simulink model "BCM2_4"  (R2021b)
settings: Solver=FixedStepDiscrete  StartTime=0.0  StopTime=1  FixedStep=0.001  RelTol=1e-3  EnableMultiTasking=on
InitFcn:
  | mbd_mpc_consistency_checks(bdroot(gcs));
model workspace (MAT data in the model file):
  CAN_rec : Simulink.Signal (value not decoded)
  CAN_transm_stat : Simulink.Signal (value not decoded)
  CAN_trm : Simulink.Signal (value not decoded)
  DITHER_CFB0 : Simulink.Parameter (value not decoded)
  DITHER_CFB1 : Simulink.Parameter (value not decoded)
  DITHER_CFB2 : Simulink.Parameter (value not decoded)
  DITHER_EN0 : Simulink.Parameter (value not decoded)
  DITHER_EN1 : Simulink.Parameter (value not decoded)
  DITHER_EN2 : Simulink.Parameter (value not decoded)
  DITHER_SIZE0 : Simulink.Parameter (value not decoded)
  DITHER_SIZE1 : Simulink.Parameter (value not decoded)
  DITHER_SIZE2 : Simulink.Parameter (value not decoded)
  DITHER_STEP0 : Simulink.Parameter (value not decoded)
  DITHER_STEP1 : Simulink.Parameter (value not decoded)
  DITHER_STEP2 : Simulink.Parameter (value not decoded)
  DITHER_SYNC0 : Simulink.Parameter (value not decoded)
  DITHER_SYNC1 : Simulink.Parameter (value not decoded)
  DITHER_SYNC2 : Simulink.Parameter (value not decoded)
  ECUMbut : Simulink.Signal (value not decoded)
  FAULTN : Simulink.Signal (value not decoded)
  FM0 : Simulink.Parameter (value not decoded)
  FM1 : Simulink.Parameter (value not decoded)
  FM2 : Simulink.Parameter (value not decoded)
  FME : Simulink.Parameter (value not decoded)
  Fsys_M : Simulink.Parameter (value not decoded)
  Fsys_N : Simulink.Parameter (value not decoded)
  Fsys_WDEN : Simulink.Parameter (value not decoded)
  Fsys_div : Simulink.Parameter (value not decoded)
  HL0 : Simulink.Parameter (value not decoded)
  HL1 : Simulink.Parameter (value not decoded)
  HL2 : Simulink.Parameter (value not decoded)
  IDIAG0 : Simulink.Parameter (value not decoded)
  IDIAG1 : Simulink.Parameter (value not decoded)
  IDIAG2 : Simulink.Parameter (value not decoded)
  Ivalve : Simulink.Signal (value not decoded)
  KI_index0 : Simulink.Parameter (value not decoded)
  KI_index1 : Simulink.Parameter (value not decoded)
  KI_index2 : Simulink.Parameter (value not decoded)
  PWM_Period0 : Simulink.Parameter (value not decoded)
  PWM_Period1 : Simulink.Parameter (value not decoded)
  PWM_Period2 : Simulink.Parameter (value not decoded)
  RESN : Simulink.Signal (value not decoded)
  SR0 : Simulink.Parameter (value not decoded)
  SR1 : Simulink.Parameter (value not decoded)
  SR2 : Simulink.Parameter (value not decoded)
  Vparam : Simulink.Signal (value not decoded)
  block_tle : Simulink.Signal (value not decoded)
  disp : Simulink.Signal (value not decoded)
  ee_adr : Simulink.Signal (value not decoded)
  ee_en_rd : Simulink.Signal (value not decoded)
  ee_en_wr : Simulink.Signal (value not decoded)
  ee_idle : Simulink.Signal (value not decoded)
  ee_read : Simulink.Signal (value not decoded)
  ee_recv : Simulink.Signal (value not decoded)
  ee_send : Simulink.Signal (value not decoded)
  in_stats : Simulink.Signal (value not decoded)
  inputs : Simulink.Signal (value not decoded)
  light : Simulink.Signal (value not decoded)
  out_drv : Simulink.Signal (value not decoded)
  out_drv_test : Simulink.Signal (value not decoded)
  out_test_en : Simulink.Signal (value not decoded)
  recv_spi2 : Simulink.Signal (value not decoded)
  ret : Simulink.Signal (value not decoded)
  spi_rcv_tle82453 : Simulink.Signal (value not decoded)
  tle82453_Ivlv : Simulink.Signal (value not decoded)
  tle82453_err : Simulink.Signal (value not decoded)
  tle82453_reset : Simulink.Signal (value not decoded)
  wtdg_CAN : Simulink.Signal (value not decoded)
symbols that are objects in the model workspace (value not decoded): CAN_rec, CAN_transm_stat, ECUMbut, inputs, Ivalve, out_drv_test, recv_spi2, ret, SR0, tle82453_Ivlv
undefined symbols (not defined in the file or in its folder): color, LQFP
libraries: simulink x68, mbd_mpc574x_ec_toolbox x50, canmsglib x42, hdlsllib x9, commutil2 x7, etargetslib x4
(part 4 of 6)

== system BCM2_4/CAN0 Transmit buf 5-21/18FEEA2F buf = 9/18FEEA2F buf = 9 ==
  Constant4 : Constant  OutDataTypeStr=boolean
  Data Store Read : DataStoreRead  DataStoreName=CAN_rec  DataStoreElements=CAN_rec.m18FEEA2F(:)  IndexOptions=Index vector (dialog)  Indices=1  OutputSizes=1
  Data Store Write : DataStoreWrite  DataStoreName=CAN_transm_stat  DataStoreElements=CAN_transm_stat(9)  IndexOptions=Index vector (dialog)  Indices=1  OutputSizes=1
  FCAN_Send : mbd_mpc574x_ec_toolbox/Communication Blocks/CAN Blocks/FCAN_Send  Priority=2  can_instance=0  can_mode=Non-blocking  can_timeout_ms=0  can_mb_idx=9  can_extended_id=on  can_is_remote=off  can_id=18FEEA2F  show_adv_opts=on  can_fd_enable=off  can_enable_brs=off  can_fd_padding=0
      settings: SourceProductName=NXP Model-Based Design Toolbox for MPC57xx MCUs
  Width : Width  DataType=uint8
  wires:
  Data Store Read/1 -> FCAN_Send/1, Width/1
  Constant4/1 -> Data Store Write/1
  Width/1 -> FCAN_Send/2

== system BCM2_4/CAN0 Transmit buf 5-21/Tx_Complete/If Action Subsystem1 ==
  Action Port : ActionPort  ActionPortLabel=case [ 7 ]:
  Constant : Constant  Value=0  OutDataTypeStr=boolean
  Data Store Write : DataStoreWrite  DataStoreName=CAN_transm_stat  DataStoreElements=CAN_transm_stat(7)  IndexOptions=Index vector (dialog)  Indices=1  OutputSizes=1
  wires:
  Constant/1 -> Data Store Write/1

== system BCM2_4/CAN0 Transmit buf 5-21/Tx_Complete/If Action Subsystem2 ==
  Action Port : ActionPort  ActionPortLabel=default:

== system BCM2_4/CAN0 Transmit buf 5-21/Tx_Complete/If Action Subsystem3 ==
  Action Port : ActionPort  ActionPortLabel=case [ 8 ]:
  Constant : Constant  Value=0  OutDataTypeStr=boolean
  Data Store Write : DataStoreWrite  DataStoreName=CAN_transm_stat  DataStoreElements=CAN_transm_stat(8)  IndexOptions=Index vector (dialog)  Indices=1  OutputSizes=1
  wires:
  Constant/1 -> Data Store Write/1

== system BCM2_4/CAN0 Transmit buf 5-21/Tx_Complete/If Action Subsystem4 ==
  Action Port : ActionPort  ActionPortLabel=case [ 9 ]:
  Constant : Constant  Value=0  OutDataTypeStr=boolean
  Data Store Write : DataStoreWrite  DataStoreName=CAN_transm_stat  DataStoreElements=CAN_transm_stat(9)  IndexOptions=Index vector (dialog)  Indices=1  OutputSizes=1
  wires:
  Constant/1 -> Data Store Write/1

== system BCM2_4/CAN0 Transmit buf 5-21/Tx_Complete/If Action Subsystem5 ==
  Action Port : ActionPort  ActionPortLabel=case [ 10 ]:
  Constant : Constant  Value=0  OutDataTypeStr=boolean
  Data Store Write : DataStoreWrite  DataStoreName=CAN_transm_stat  DataStoreElements=CAN_transm_stat(10)  IndexOptions=Index vector (dialog)  Indices=1  OutputSizes=1
  wires:
  Constant/1 -> Data Store Write/1

== system BCM2_4/CAN0 Transmit buf 5-21/Tx_Complete/If Action Subsystem6 ==
  Action Port : ActionPort  ActionPortLabel=case [ 11 ]:
  Constant : Constant  Value=0  OutDataTypeStr=boolean
  Data Store Write : DataStoreWrite  DataStoreName=CAN_transm_stat  DataStoreElements=CAN_transm_stat(11)  IndexOptions=Index vector (dialog)  Indices=1  OutputSizes=1
  wires:
  Constant/1 -> Data Store Write/1

== system BCM2_4/CAN0 Transmit buf 5-21/Tx_Complete/If Action Subsystem7 ==
  Action Port : ActionPort  ActionPortLabel=case [ 6 ]:
  Constant : Constant  Value=0  OutDataTypeStr=boolean
  Data Store Write : DataStoreWrite  DataStoreName=CAN_transm_stat  DataStoreElements=CAN_transm_stat(6)  IndexOptions=Index vector (dialog)  Indices=1  OutputSizes=1
  wires:
  Constant/1 -> Data Store Write/1

== system BCM2_4/CAN0 Transmit buf 5-21/Tx_Complete/If Action Subsystem8 ==
  Action Port : ActionPort  ActionPortLabel=case [ 5 ]:
  Constant : Constant  Value=0  OutDataTypeStr=boolean
  Data Store Write : DataStoreWrite  DataStoreName=CAN_transm_stat  DataStoreElements=CAN_transm_stat(5)  IndexOptions=Index vector (dialog)  Indices=1  OutputSizes=1
  wires:
  Constant/1 -> Data Store Write/1

== system BCM2_4/CAN1 Transmit buf 27-43/Tx_Complete/If Action Subsystem1 ==
  Action Port : ActionPort  ActionPortLabel=case [ 29 ]:
  Constant : Constant  Value=0  OutDataTypeStr=boolean
  Data Store Write : DataStoreWrite  DataStoreName=CAN_transm_stat  DataStoreElements=CAN_transm_stat(29)  IndexOptions=Index vector (dialog)  Indices=1  OutputSizes=1
  wires:
  Constant/1 -> Data Store Write/1

== system BCM2_4/CAN1 Transmit buf 27-43/Tx_Complete/If Action Subsystem2 ==
  Action Port : ActionPort  ActionPortLabel=default:

== system BCM2_4/CAN1 Transmit buf 27-43/Tx_Complete/If Action Subsystem3 ==
  Action Port : ActionPort  ActionPortLabel=case [ 30 ]:
  Constant : Constant  Value=0  OutDataTypeStr=boolean
  Data Store Write : DataStoreWrite  DataStoreName=CAN_transm_stat  DataStoreElements=CAN_transm_stat(30)  IndexOptions=Index vector (dialog)  Indices=1  OutputSizes=1
  wires:
  Constant/1 -> Data Store Write/1

== system BCM2_4/CAN1 Transmit buf 27-43/Tx_Complete/If Action Subsystem4 ==
  Action Port : ActionPort  ActionPortLabel=case [ 31 ]:
  Constant : Constant  Value=0  OutDataTypeStr=boolean
  Data Store Write : DataStoreWrite  DataStoreName=CAN_transm_stat  DataStoreElements=CAN_transm_stat(31)  IndexOptions=Index vector (dialog)  Indices=1  OutputSizes=1
  wires:
  Constant/1 -> Data Store Write/1

== system BCM2_4/CAN1 Transmit buf 27-43/Tx_Complete/If Action Subsystem7 ==
  Action Port : ActionPort  ActionPortLabel=case [ 28 ]:
  Constant : Constant  Value=0  OutDataTypeStr=boolean
  Data Store Write : DataStoreWrite  DataStoreName=CAN_transm_stat  DataStoreElements=CAN_transm_stat(28)  IndexOptions=Index vector (dialog)  Indices=1  OutputSizes=1
  wires:
  Constant/1 -> Data Store Write/1

== system BCM2_4/CAN1 Transmit buf 27-43/Tx_Complete/If Action Subsystem8 ==
  Action Port : ActionPort  ActionPortLabel=case [ 27 ]:
  Constant : Constant  Value=0  OutDataTypeStr=boolean
  Data Store Write : DataStoreWrite  DataStoreName=CAN_transm_stat  DataStoreElements=CAN_transm_stat(27)  IndexOptions=Index vector (dialog)  Indices=1  OutputSizes=1
  wires:
  Constant/1 -> Data Store Write/1

== system BCM2_4/CAN1 Transmit buf 27-43/Активация клавиатуры buf = 27/Активация клавиатуры buf = 27 ==
  Constant : Constant  Value=[1 0 0 0 0 0 0 0]  OutDataTypeStr=uint8
  Constant4 : Constant  OutDataTypeStr=boolean
  Data Store Write : DataStoreWrite  DataStoreName=CAN_transm_stat  DataStoreElements=CAN_transm_stat(27)  IndexOptions=Index vector (dialog)  Indices=1  OutputSizes=1
  FCAN_Send : mbd_mpc574x_ec_toolbox/Communication Blocks/CAN Blocks/FCAN_Send  Priority=2  can_instance=1  can_mode=Non-blocking  can_timeout_ms=0  can_mb_idx=27  can_extended_id=off  can_is_remote=off  can_id=0  show_adv_opts=on  can_fd_enable=off  can_enable_brs=off  can_fd_padding=0
      settings: SourceProductName=NXP Model-Based Design Toolbox for MPC57xx MCUs
  Width : Width  DataType=uint8
  wires:
  Constant4/1 -> Data Store Write/1
  Width/1 -> FCAN_Send/2
  Constant/1 -> Width/1, FCAN_Send/1

== system BCM2_4/CAN1 Transmit buf 27-43/Цвет клавиатуры 12 buf = 28/Цвет клавиатуры buf = 28 ==
  Chart : Stateflow chart  TreatAsAtomicUnit=on
  Constant4 : Constant  OutDataTypeStr=boolean
  Data Store Read : DataStoreRead  DataStoreName=ECUMbut  DataStoreElements=ECUMbut.color12(:)  IndexOptions=Index vector (dialog)  Indices=1  OutputSizes=1
  Data Store Write : DataStoreWrite  DataStoreName=CAN_transm_stat  DataStoreElements=CAN_transm_stat(28)  IndexOptions=Index vector (dialog)  Indices=1  OutputSizes=1
  FCAN_Send : mbd_mpc574x_ec_toolbox/Communication Blocks/CAN Blocks/FCAN_Send  Priority=2  can_instance=1  can_mode=Non-blocking  can_timeout_ms=0  can_mb_idx=28  can_extended_id=off  can_is_remote=off  can_id=215  show_adv_opts=on  can_fd_enable=off  can_enable_brs=off  can_fd_padding=0
      settings: SourceProductName=NXP Model-Based Design Toolbox for MPC57xx MCUs
  Width : Width  DataType=uint8
  wires:
  Width/1 -> FCAN_Send/2
  Constant4/1 -> Data Store Write/1
  Data Store Read/1 -> Chart/1(input)
  Chart/1(out) -> Width/1, FCAN_Send/1

== system BCM2_4/CAN1 Transmit buf 27-43/Цвет клавиатуры 4 buf = 30/Цвет клавиатуры buf = 30 ==
  Chart : Stateflow chart  TreatAsAtomicUnit=on
  Constant4 : Constant  OutDataTypeStr=boolean
  Data Store Read : DataStoreRead  DataStoreName=ECUMbut  DataStoreElements=ECUMbut.color4(:)  IndexOptions=Index vector (dialog)  Indices=1  OutputSizes=1
  Data Store Write : DataStoreWrite  DataStoreName=CAN_transm_stat  DataStoreElements=CAN_transm_stat(30)  IndexOptions=Index vector (dialog)  Indices=1  OutputSizes=1
  FCAN_Send : mbd_mpc574x_ec_toolbox/Communication Blocks/CAN Blocks/FCAN_Send  Priority=2  can_instance=1  can_mode=Non-blocking  can_timeout_ms=0  can_mb_idx=30  can_extended_id=off  can_is_remote=off  can_id=212  show_adv_opts=on  can_fd_enable=off  can_enable_brs=off  can_fd_padding=0
      settings: SourceProductName=NXP Model-Based Design Toolbox for MPC57xx MCUs
  Width : Width  DataType=uint8
  wires:
  Chart/1(out) -> FCAN_Send/1, Width/1
  Data Store Read/1 -> Chart/1(input)
  Constant4/1 -> Data Store Write/1
  Width/1 -> FCAN_Send/2

== system BCM2_4/CAN1 Transmit buf 27-43/подсветка клавиатуры buf = 29/подсветка клавиатуры buf = 29 ==
  Chart : Stateflow chart  TreatAsAtomicUnit=on
  Constant4 : Constant  OutDataTypeStr=boolean
  Data Store Write : DataStoreWrite  DataStoreName=CAN_transm_stat  DataStoreElements=CAN_transm_stat(29)  IndexOptions=Index vector (dialog)  Indices=1  OutputSizes=1
  FCAN_Send : mbd_mpc574x_ec_toolbox/Communication Blocks/CAN Blocks/FCAN_Send  Priority=2  can_instance=1  can_mode=Non-blocking  can_timeout_ms=0  can_mb_idx=29  can_extended_id=off  can_is_remote=off  can_id=615  show_adv_opts=on  can_fd_enable=off  can_enable_brs=off  can_fd_padding=0
      settings: SourceProductName=NXP Model-Based Design Toolbox for MPC57xx MCUs
  Width : Width  DataType=uint8
  wires:
  Constant4/1 -> Data Store Write/1
  Width/1 -> FCAN_Send/2
  Chart/1(out) -> FCAN_Send/1, Width/1

== system BCM2_4/CAN1 Transmit buf 27-43/подсветка клавиатуры buf = 31/подсветка клавиатуры buf = 31 ==
  Chart : Stateflow chart  TreatAsAtomicUnit=on
  Constant1 : Constant  OutDataTypeStr=boolean
  Data Store Write1 : DataStoreWrite  DataStoreName=CAN_transm_stat  DataStoreElements=CAN_transm_stat(31)  IndexOptions=Index vector (dialog)  Indices=1  OutputSizes=1
  FCAN_Send : mbd_mpc574x_ec_toolbox/Communication Blocks/CAN Blocks/FCAN_Send  Priority=2  can_instance=1  can_mode=Non-blocking  can_timeout_ms=0  can_mb_idx=31  can_extended_id=off  can_is_remote=off  can_id=612  show_adv_opts=on  can_fd_enable=off  can_enable_brs=off  can_fd_padding=0
      settings: SourceProductName=NXP Model-Based Design Toolbox for MPC57xx MCUs
  Width : Width  DataType=uint8
  wires:
  Constant1/1 -> Data Store Write1/1
  Chart/1(out) -> Width/1, FCAN_Send/1
  Width/1 -> FCAN_Send/2

== system BCM2_4/CAN2 Transmit buf 49-59/EBC1 0x18F0010D Педаль тормоза buf = 9/EBC1 0x18F0010D buf = 9 ==
  Constant : Constant  Value=[1 2 3 4 5 6 7 8]  OutDataTypeStr=uint8
  Constant4 : Constant  OutDataTypeStr=boolean
  Data Store Write : DataStoreWrite  DataStoreName=CAN_transm_stat  DataStoreElements=CAN_transm_stat(9)  IndexOptions=Index vector (dialog)  Indices=1  OutputSizes=1
  FCAN_Send : mbd_mpc574x_ec_toolbox/Communication Blocks/CAN Blocks/FCAN_Send  Priority=2  can_instance=2  can_mode=Non-blocking  can_timeout_ms=0  can_mb_idx=9  can_extended_id=on  can_is_remote=off  can_id=18F0010D  show_adv_opts=on  can_fd_enable=off  can_enable_brs=off  can_fd_padding=0
      settings: SourceProductName=NXP Model-Based Design Toolbox for MPC57xx MCUs
  Width : Width  DataType=uint8
  wires:
  Constant/1 -> FCAN_Send/1, Width/1
  Width/1 -> FCAN_Send/2
  Constant4/1 -> Data Store Write/1

== system BCM2_4/CAN2 Transmit buf 49-59/Tx_Complete/If Action Subsystem2 ==
  Action Port : ActionPort  ActionPortLabel=default:

== system BCM2_4/CAN2 Transmit buf 49-59/Tx_Complete/If Action Subsystem7 ==
  Action Port : ActionPort  ActionPortLabel=case [ 21 ]:

== system BCM2_4/CAN2 Transmit buf 49-59/Tx_Complete/If Action Subsystem8 ==
  Action Port : ActionPort  ActionPortLabel=case [ 9 ]:
  Constant : Constant  Value=0  OutDataTypeStr=boolean
  Data Store Write : DataStoreWrite  DataStoreName=CAN_transm_stat  DataStoreElements=CAN_transm_stat(9)  IndexOptions=Index vector (dialog)  Indices=1  OutputSizes=1
  wires:
  Constant/1 -> Data Store Write/1

== system BCM2_4/CAN_Receive/RX_FIFO_Complete_Event buf 0-4/0CFxxxxx reinit buf0 ==
  Action Port : ActionPort  ActionPortLabel=case [ 0 ]:
  FCAN_Receive_ID_0CFxxxxx : mbd_mpc574x_ec_toolbox/Communication Blocks/CAN Blocks/FCAN_Receive  can_instance=0  can_mode=Non-blocking  can_timeout_ms=0  can_mb_idx=0  can_extended_id=on  can_is_remote=off  can_id=0CF00000  can_msg_mask=FFF00000  show_adv_opts=off  can_use_rxfifo=off  can_fd_enable=off
      settings: SourceProductName=NXP Model-Based Design Toolbox for MPC57xx MCUs

== system BCM2_4/CAN_Receive/RX_FIFO_Complete_Event buf 0-4/1811xxxx reinit buf2 ==
  Action Port : ActionPort  ActionPortLabel=case [ 2 ]:
  FCAN_Receive_ID_1811xxxxx : mbd_mpc574x_ec_toolbox/Communication Blocks/CAN Blocks/FCAN_Receive  can_instance=0  can_mode=Non-blocking  can_timeout_ms=0  can_mb_idx=2  can_extended_id=on  can_is_remote=off  can_id=18110000  can_msg_mask=FFFF0000  show_adv_opts=off  can_use_rxfifo=off  can_fd_enable=off
      settings: SourceProductName=NXP Model-Based Design Toolbox for MPC57xx MCUs

== system BCM2_4/CAN_Receive/RX_FIFO_Complete_Event buf 0-4/18Fxxxxx reinit buf1 ==
  Action Port : ActionPort  ActionPortLabel=case [ 1 ]:
  FCAN_Receive_ID_18Fxxxxx : mbd_mpc574x_ec_toolbox/Communication Blocks/CAN Blocks/FCAN_Receive  can_instance=0  can_mode=Non-blocking  can_timeout_ms=0  can_mb_idx=1  can_extended_id=on  can_is_remote=off  can_id=18F00000  can_msg_mask=FFF00000  show_adv_opts=off  can_use_rxfifo=off  can_fd_enable=off
      settings: SourceProductName=NXP Model-Based Design Toolbox for MPC57xx MCUs

== system BCM2_4/CAN_Receive/RX_FIFO_Complete_Event buf 0-4/1FEEF888 reinit buf3 ==
  Action Port : ActionPort  ActionPortLabel=case [ 3 ]:
  FCAN_Receive_ID_1FEEF888 : mbd_mpc574x_ec_toolbox/Communication Blocks/CAN Blocks/FCAN_Receive  can_instance=0  can_mode=Non-blocking  can_timeout_ms=0  can_mb_idx=3  can_extended_id=on  can_is_remote=off  can_id=1FEEF888  can_msg_mask=FFFFFFFF  show_adv_opts=off  can_use_rxfifo=off  can_fd_enable=off
      settings: SourceProductName=NXP Model-Based Design Toolbox for MPC57xx MCUs

== system BCM2_4/CAN_Receive/RX_FIFO_Complete_Event buf 0-4/CCVS1 0x18FEF100 buf = 1 Vspd ==
  Data : Inport
  Action Port : ActionPort  ActionPortLabel=case [ 419361024 ]:
  CAN Pack : canmsglib/CAN Pack  CANdbFile=C:\Documents\Документация\J1939\j1939.dbc  MsgList=A1  MsgName=CANPACK  MsgIDType=Extended (29-bit identifier)  MsgIdentifier=hex2dec('18FEF100')  MsgLength=8  Remote=off  ApplyMinMax=off  BusOutput=off  SignalInfo={ 'ActualEngPercentTorque', '16', '8', 'LE', 'unsigned', 'Standard', '0', '1', '-125', '-125', '125'; 'DriversDemandEngPercentTorque', '8', '8', 'LE', 'unsigned', 'Standard', '0', '1', '-125', '-125', '125'; 'EngDemandPercentTorque', '56', '8', 'LE', 'unsigned', 'Standard', '0', '1', '-125', '-125', '125'; 'EngSpeed', '24', '16', 'LE', 'unsigned', 'Standard', '0', '0.125', '0', '0', '8031.875'; 'EngStarterMode', '48', '4', 'LE', 'unsigned', 'Standard', '0', '1', '0', '0', '15'; 'EngTorqueMode', '0', '4', 'LE', 'unsigned', 'Standard', '0', '1', '0', '0', '15'; 'SrcAddrssOfCtrllngDvcForEngCtrl', '40', '8', 'LE', 'unsigned', 'Standard', '0', '1', '0', '0', '255' }
      settings: SourceProductBaseCode=ME,XP,VN  DataFormat=raw data
  CAN Unpack1 : canmsglib/CAN Unpack  CANdbFile=C:\Users\km-rta\Desktop\engineering\j1939.dbc  MsgList=A1  MsgName=CCVS1  MsgIDType=Extended (29-bit identifier)  MsgIdentifier=hex2dec('18FEF100')  MsgLength=8  SignalInfo={ 'WheelBasedVehicleSpeed', '8', '16', 'LE', 'unsigned', 'Standard', '0', '3.906250e-03', '0', '0', '2.509960e+02' }  IDPort=off  TimestampPort=off  ErrorPort=off  RemotePort=off  LengthPort=off  StatusPort=off  ApplyMinMax=off
      settings: SourceProductName=Simulink Real-Time
  Constant : Constant  Value=0  OutDataTypeStr=uint16
  Data Store Write1 : DataStoreWrite  DataStoreName=wtdg_CAN  DataStoreElements=wtdg_CAN.CCVS1_00  IndexOptions=Index vector (dialog)  Indices=1  OutputSizes=1
  Data Store Write4 : DataStoreWrite  DataStoreName=Vparam  DataStoreElements=Vparam.Vspd  IndexOptions=Index vector (dialog)  Indices=1  OutputSizes=1
  wires:
  Data/1 -> CAN Pack/1
  CAN Unpack1/1 -> Data Store Write4/1
  CAN Pack/1 -> CAN Unpack1/1
  Constant/1 -> Data Store Write1/1

== system BCM2_4/CAN_Receive/RX_FIFO_Complete_Event buf 0-4/EBC1 0x18F0010B buf = 1 Brake pos ==
  Data : Inport
  Action Port : ActionPort  ActionPortLabel=case [ 418382091 ]:
  CAN Pack : canmsglib/CAN Pack  CANdbFile=C:\Documents\Документация\J1939\j1939.dbc  MsgList=A1  MsgName=CANPACK  MsgIDType=Extended (29-bit identifier)  MsgIdentifier=hex2dec('18F0010B')  MsgLength=8  Remote=off  ApplyMinMax=off  BusOutput=off  SignalInfo={ 'ActualEngPercentTorque', '16', '8', 'LE', 'unsigned', 'Standard', '0', '1', '-125', '-125', '125'; 'DriversDemandEngPercentTorque', '8', '8', 'LE', 'unsigned', 'Standard', '0', '1', '-125', '-125', '125'; 'EngDemandPercentTorque', '56', '8', 'LE', 'unsigned', 'Standard', '0', '1', '-125', '-125', '125'; 'EngSpeed', '24', '16', 'LE', 'unsigned', 'Standard', '0', '0.125', '0', '0', '8031.875'; 'EngStarterMode', '48', '4', 'LE', 'unsigned', 'Standard', '0', '1', '0', '0', '15'; 'EngTorqueMode', '0', '4', 'LE', 'unsigned', 'Standard', '0', '1', '0', '0', '15'; 'SrcAddrssOfCtrllngDvcForEngCtrl', '40', '8', 'LE', 'unsigned', 'Standard', '0', '1', '0', '0', '255' }
      settings: SourceProductBaseCode=ME,XP,VN  DataFormat=raw data
  CAN Unpack3 : canmsglib/CAN Unpack  CANdbFile=C:\Users\km-rta\Desktop\engineering\j1939.dbc  MsgList=EBC1  MsgName=EBC1  MsgIDType=Extended (29-bit identifier)  MsgIdentifier=hex2dec('18F0010B')  MsgLength=8  SignalInfo={ 'BrakePedalPos', '8', '8', 'LE', 'unsigned', 'Standard', '0', '4.000000e-01', '0', '0', '100' }  IDPort=off  TimestampPort=off  ErrorPort=off  RemotePort=off  LengthPort=off  StatusPort=off  ApplyMinMax=off
      settings: SourceProductBaseCode=ME,XP,VN
  Constant : Constant  Value=0  OutDataTypeStr=uint16
  Data Store Write : DataStoreWrite  DataStoreName=Vparam  DataStoreElements=Vparam.BrakePos  IndexOptions=Index vector (dialog)  Indices=1  OutputSizes=1
  Data Store Write1 : DataStoreWrite  DataStoreName=wtdg_CAN  DataStoreElements=wtdg_CAN.EBC1  IndexOptions=Index vector (dialog)  Indices=1  OutputSizes=1
  Data Type Conversion : DataTypeConversion  OutDataTypeStr=uint8
  wires:
  CAN Pack/1 -> CAN Unpack3/1
  Data/1 -> CAN Pack/1
  CAN Unpack3/1 -> Data Type Conversion/1
  Constant/1 -> Data Store Write1/1
  Data Type Conversion/1 -> Data Store Write/1

== system BCM2_4/CAN_Receive/RX_FIFO_Complete_Event buf 0-4/EEC1 0x0CF00300 buf = 0 Pedal pos ==
  Data : Inport
  Action Port : ActionPort  ActionPortLabel=case [ 217056000 ]:
  CAN Pack : canmsglib/CAN Pack  CANdbFile=C:\Documents\Документация\J1939\j1939.dbc  MsgList=A1  MsgName=CANPACK  MsgIDType=Extended (29-bit identifier)  MsgIdentifier=hex2dec('0CF00300')  MsgLength=8  Remote=off  ApplyMinMax=off  BusOutput=off  SignalInfo={ 'ActualEngPercentTorque', '16', '8', 'LE', 'unsigned', 'Standard', '0', '1', '-125', '-125', '125'; 'DriversDemandEngPercentTorque', '8', '8', 'LE', 'unsigned', 'Standard', '0', '1', '-125', '-125', '125'; 'EngDemandPercentTorque', '56', '8', 'LE', 'unsigned', 'Standard', '0', '1', '-125', '-125', '125'; 'EngSpeed', '24', '16', 'LE', 'unsigned', 'Standard', '0', '0.125', '0', '0', '8031.875'; 'EngStarterMode', '48', '4', 'LE', 'unsigned', 'Standard', '0', '1', '0', '0', '15'; 'EngTorqueMode', '0', '4', 'LE', 'unsigned', 'Standard', '0', '1', '0', '0', '15'; 'SrcAddrssOfCtrllngDvcForEngCtrl', '40', '8', 'LE', 'unsigned', 'Standard', '0', '1', '0', '0', '255' }
      settings: SourceProductBaseCode=ME,XP,VN  DataFormat=raw data
  CAN Unpack5 : canmsglib/CAN Unpack  CANdbFile=C:\Users\km-rta\Desktop\engineering\j1939.dbc  MsgList=EEC1  MsgName=EEC1  MsgIDType=Extended (29-bit identifier)  MsgIdentifier=hex2dec('0CF00300')  MsgLength=8  SignalInfo={ 'DriversDemandEngPercentTorque', '8', '8', 'LE', 'unsigned', 'Standard', '0', '0.4', '0', '0', '102' }  IDPort=off  TimestampPort=off  ErrorPort=off  RemotePort=off  LengthPort=off  StatusPort=off  ApplyMinMax=off
      settings: SourceProductBaseCode=ME,XP,VN
  Constant : Constant  Value=0  OutDataTypeStr=uint16
  Data Store Write : DataStoreWrite  DataStoreName=Vparam  DataStoreElements=Vparam.PedalPos  IndexOptions=Index vector (dialog)  Indices=1  OutputSizes=1
  Data Store Write1 : DataStoreWrite  DataStoreName=wtdg_CAN  DataStoreElements=wtdg_CAN.EEC1_300  IndexOptions=Index vector (dialog)  Indices=1  OutputSizes=1
  Data Type Conversion : DataTypeConversion  OutDataTypeStr=uint8
  wires:
  Constant/1 -> Data Store Write1/1
  CAN Unpack5/1 -> Data Type Conversion/1
  CAN Pack/1 -> CAN Unpack5/1
  Data/1 -> CAN Pack/1
  Data Type Conversion/1 -> Data Store Write/1

== system BCM2_4/CAN_Receive/RX_FIFO_Complete_Event buf 0-4/EEC1 0x0CF00400 buf = 0 Espd ==
  Data : Inport
  Action Port : ActionPort  ActionPortLabel=case [ 217056256 ]:
  CAN Pack : canmsglib/CAN Pack  CANdbFile=C:\Documents\Документация\J1939\j1939.dbc  MsgList=A1  MsgName=CANPACK  MsgIDType=Extended (29-bit identifier)  MsgIdentifier=hex2dec('0CF00400')  MsgLength=8  Remote=off  ApplyMinMax=off  BusOutput=off  SignalInfo={ 'ActualEngPercentTorque', '16', '8', 'LE', 'unsigned', 'Standard', '0', '1', '-125', '-125', '125'; 'DriversDemandEngPercentTorque', '8', '8', 'LE', 'unsigned', 'Standard', '0', '1', '-125', '-125', '125'; 'EngDemandPercentTorque', '56', '8', 'LE', 'unsigned', 'Standard', '0', '1', '-125', '-125', '125'; 'EngSpeed', '24', '16', 'LE', 'unsigned', 'Standard', '0', '0.125', '0', '0', '8031.875'; 'EngStarterMode', '48', '4', 'LE', 'unsigned', 'Standard', '0', '1', '0', '0', '15'; 'EngTorqueMode', '0', '4', 'LE', 'unsigned', 'Standard', '0', '1', '0', '0', '15'; 'SrcAddrssOfCtrllngDvcForEngCtrl', '40', '8', 'LE', 'unsigned', 'Standard', '0', '1', '0', '0', '255' }
      settings: SourceProductBaseCode=ME,XP,VN  DataFormat=raw data
  CAN Unpack5 : canmsglib/CAN Unpack  CANdbFile=C:\Users\km-rta\Desktop\engineering\j1939.dbc  MsgList=EEC1  MsgName=EEC1  MsgIDType=Extended (29-bit identifier)  MsgIdentifier=hex2dec('0CF00400')  MsgLength=8  SignalInfo={ 'EngSpeed', '24', '16', 'LE', 'unsigned', 'Standard', '0', '1.250000e-01', '0', '0', '8.031875e+03' }  IDPort=off  TimestampPort=off  ErrorPort=off  RemotePort=off  LengthPort=off  StatusPort=off  ApplyMinMax=off
      settings: SourceProductBaseCode=ME,XP,VN
  Constant : Constant  Value=0  OutDataTypeStr=uint16
  Data Store Write : DataStoreWrite  DataStoreName=Vparam  DataStoreElements=Vparam.Espd  IndexOptions=Index vector (dialog)  Indices=1  OutputSizes=1
  Data Store Write1 : DataStoreWrite  DataStoreName=wtdg_CAN  DataStoreElements=wtdg_CAN.EEC1_400  IndexOptions=Index vector (dialog)  Indices=1  OutputSizes=1
  Data Type Conversion : DataTypeConversion  OutDataTypeStr=uint16
  wires:
  Data/1 -> CAN Pack/1
  CAN Pack/1 -> CAN Unpack5/1
  CAN Unpack5/1 -> Data Type Conversion/1
  Constant/1 -> Data Store Write1/1
  Data Type Conversion/1 -> Data Store Write/1

== system BCM2_4/CAN_Receive/RX_FIFO_Complete_Event buf 0-4/EEPROM R//W 0x18FEF460 buf = 1 EEPROM ==
  Data : Inport
  Action Port : ActionPort  ActionPortLabel=case [ 419361888 ]:
  CAN Pack : canmsglib/CAN Pack  CANdbFile=C:\Documents\Документация\J1939\j1939.dbc  MsgList=A1  MsgName=CANPACK  MsgIDType=Extended (29-bit identifier)  MsgIdentifier=hex2dec('18FEF460')  MsgLength=8  Remote=off  ApplyMinMax=off  BusOutput=off  SignalInfo={ 'ActualEngPercentTorque', '16', '8', 'LE', 'unsigned', 'Standard', '0', '1', '-125', '-125', '125'; 'DriversDemandEngPercentTorque', '8', '8', 'LE', 'unsigned', 'Standard', '0', '1', '-125', '-125', '125'; 'EngDemandPercentTorque', '56', '8', 'LE', 'unsigned', 'Standard', '0', '1', '-125', '-125', '125'; 'EngSpeed', '24', '16', 'LE', 'unsigned', 'Standard', '0', '0.125', '0', '0', '8031.875'; 'EngStarterMode', '48', '4', 'LE', 'unsigned', 'Standard', '0', '1', '0', '0', '15'; 'EngTorqueMode', '0', '4', 'LE', 'unsigned', 'Standard', '0', '1', '0', '0', '15'; 'SrcAddrssOfCtrllngDvcForEngCtrl', '40', '8', 'LE', 'unsigned', 'Standard', '0', '1', '0', '0', '255' }
      settings: SourceProductBaseCode=ME,XP,VN  DataFormat=raw data
  CAN Unpack1 : canmsglib/CAN Unpack  CANdbFile=C:\Users\km-rta\Desktop\engineering\j1939.dbc  MsgList=A1  MsgName=EEPROM_RW  MsgIDType=Extended (29-bit identifier)  MsgIdentifier=hex2dec('18FEF460')  MsgLength=8  SignalInfo={ 'CMD', '0', '8', 'LE', 'unsigned', 'Standard', '0', '1', '0', '-Inf', 'Inf'; 'Adress', '8', '8', 'LE', 'unsigned', 'Standard', '0', '1', '0', '-Inf', 'Inf'; 'Data', '16', '16', 'LE', 'unsigned', 'Standard', '0', '1', '0', '-Inf', 'Inf' }  IDPort=off  TimestampPort=off  ErrorPort=off  RemotePort=off  LengthPort=off  StatusPort=off  ApplyMinMax=off
      settings: SourceProductName=Simulink Real-Time
  Constant : Constant  Value=0  OutDataTypeStr=uint16
  Constant1 : Constant  OutDataTypeStr=boolean
  Data Store Write1 : DataStoreWrite  DataStoreName=wtdg_CAN  DataStoreElements=wtdg_CAN.ee_wr  IndexOptions=Index vector (dialog)  Indices=1  OutputSizes=1
  Data Store Write2 : DataStoreWrite  DataStoreName=CAN_rec  DataStoreElements=CAN_rec.ee_rec_stat  IndexOptions=Index vector (dialog)  Indices=1  OutputSizes=1
  Data Store Write4 : DataStoreWrite  DataStoreName=CAN_rec  DataStoreElements=CAN_rec.ee_cmd#CAN_rec.ee_adr#CAN_rec.ee_data  IndexOptions=Index vector (dialog)  Indices=1  OutputSizes=1
  wires:
  Constant/1 -> Data Store Write1/1
  CAN Pack/1 -> CAN Unpack1/1
  Data/1 -> CAN Pack/1
  Constant1/1 -> Data Store Write2/1
  CAN Unpack1/1 -> Data Store Write4/1
  CAN Unpack1/2 -> Data Store Write4/2
  CAN Unpack1/3 -> Data Store Write4/3

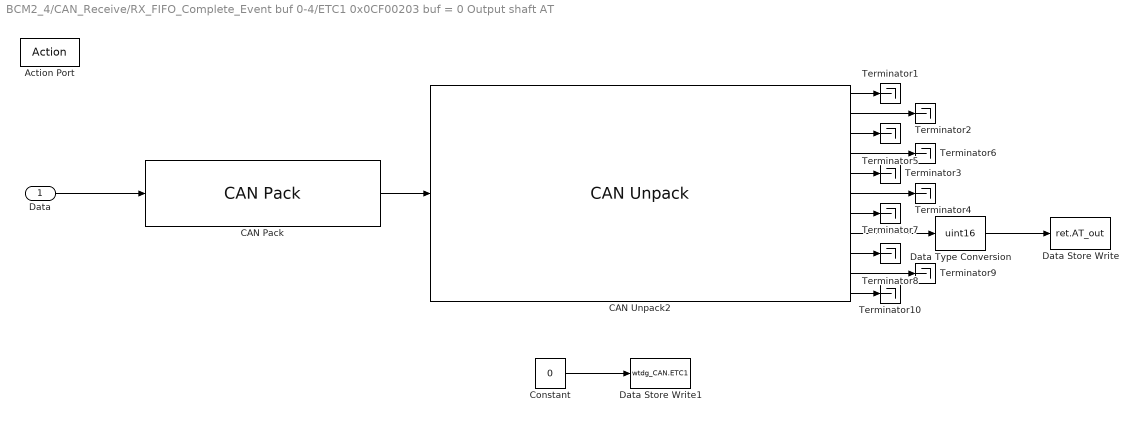
== system BCM2_4/CAN_Receive/RX_FIFO_Complete_Event buf 0-4/ETC1 0x0CF00203 buf = 0 Output shaft AT ==
  Data : Inport
  Action Port : ActionPort  ActionPortLabel=case [ 217055747 ]:
  CAN Pack : canmsglib/CAN Pack  CANdbFile=C:\Documents\Документация\J1939\j1939.dbc  MsgList=A1  MsgName=CANPACK  MsgIDType=Extended (29-bit identifier)  MsgIdentifier=hex2dec('0CF00203')  MsgLength=8  Remote=off  ApplyMinMax=off  BusOutput=off  SignalInfo={ 'ActualEngPercentTorque', '16', '8', 'LE', 'unsigned', 'Standard', '0', '1', '-125', '-125', '125'; 'DriversDemandEngPercentTorque', '8', '8', 'LE', 'unsigned', 'Standard', '0', '1', '-125', '-125', '125'; 'EngDemandPercentTorque', '56', '8', 'LE', 'unsigned', 'Standard', '0', '1', '-125', '-125', '125'; 'EngSpeed', '24', '16', 'LE', 'unsigned', 'Standard', '0', '0.125', '0', '0', '8031.875'; 'EngStarterMode', '48', '4', 'LE', 'unsigned', 'Standard', '0', '1', '0', '0', '15'; 'EngTorqueMode', '0', '4', 'LE', 'unsigned', 'Standard', '0', '1', '0', '0', '15'; 'SrcAddrssOfCtrllngDvcForEngCtrl', '40', '8', 'LE', 'unsigned', 'Standard', '0', '1', '0', '0', '255' }
      settings: SourceProductBaseCode=ME,XP,VN  DataFormat=raw data
  CAN Unpack2 : canmsglib/CAN Unpack  CANdbFile=C:\Users\km-rta\Desktop\engineering\j1939.dbc  MsgList=ETC1  MsgName=ETC1  MsgIDType=Extended (29-bit identifier)  MsgIdentifier=hex2dec('0CF00203')  MsgLength=8  SignalInfo={ 'EngMomentaryOverspeedEnable', '32', '2', 'LE', 'unsigned', 'Standard', '0', '1', '0', '0', '3'; 'MomentaryEngMaxPowerEnable', '36', '2', 'LE', 'unsigned', 'Standard', '0', '1', '0', '0', '3'; 'PercentClutchSlip', '24', '8', 'LE', 'unsigned', 'Standard', '0', '0.4', '0', '0', '100'; 'ProgressiveShiftDisable', '34', '2', 'LE', 'unsigned', 'Standard', '0', '1', '0', '0', '3'; 'SrcAddrssOfCntrllngDvcFrTrnsCtrl', '56', '8', 'LE', 'unsigned', 'Standard', '0', '1', '0', '0', '253'; 'TransDrivelineEngaged', '0', '2', 'LE', 'unsigned', 'Standard', '0', '1', '0', '0', '3'; 'TransInputShaftSpeed', '40', '16', 'LE', 'unsigned', 'Standard', '0', '0.125', '0', '0', '8031.875'; 'TransOutputShaftSpeed', '8', '16', 'LE', 'unsigned', 'Standard', '0', '0.125', '0', '0', '8031.875'; 'TransShiftInProcess', '4', '2', 'LE', 'unsigned', 'Standard', '0', '1', '0', '0', '3'; 'TrnsTorqueConverterLockupEngaged', '2', '2', 'LE', 'unsigned', 'Standard', '0', '1', '0', '0', '3'; 'TrnsTrqCnvrtrLckpTrnstnInProcess', '6', '2', 'LE', 'unsigned', 'Standard', '0', '1', '0', '0', '3' }  IDPort=off  TimestampPort=off  ErrorPort=off  RemotePort=off  LengthPort=off  StatusPort=off  ApplyMinMax=off
      settings: SourceProductName=Simulink Real-Time
  Constant : Constant  Value=0  OutDataTypeStr=uint16
  Data Store Write : DataStoreWrite  DataStoreName=ret  DataStoreElements=ret.AT_out  IndexOptions=Index vector (dialog)  Indices=1  OutputSizes=1
  Data Store Write1 : DataStoreWrite  DataStoreName=wtdg_CAN  DataStoreElements=wtdg_CAN.ETC1  IndexOptions=Index vector (dialog)  Indices=1  OutputSizes=1
  Data Type Conversion : DataTypeConversion  OutDataTypeStr=uint16
  Terminator{1..10} (10 alike) : Terminator
  wires:
  Data/1 -> CAN Pack/1
  CAN Pack/1 -> CAN Unpack2/1
  CAN Unpack2/4 -> Terminator6/1
  CAN Unpack2/3 -> Terminator5/1
  Constant/1 -> Data Store Write1/1
  CAN Unpack2/8 -> Data Type Conversion/1
  CAN Unpack2/2 -> Terminator2/1
  CAN Unpack2/1 -> Terminator1/1
  CAN Unpack2/5 -> Terminator3/1
  CAN Unpack2/6 -> Terminator4/1
  CAN Unpack2/7 -> Terminator7/1
  CAN Unpack2/9 -> Terminator8/1
  CAN Unpack2/10 -> Terminator9/1
  CAN Unpack2/11 -> Terminator10/1
  Data Type Conversion/1 -> Data Store Write/1

== system BCM2_4/CAN_Receive/RX_FIFO_Complete_Event buf 0-4/RF 0x18FEFB10 buf = 1 Ret temp ==
  Data : Inport
  Action Port : ActionPort  ActionPortLabel=case [ 419363600 ]:
  CAN Pack : canmsglib/CAN Pack  CANdbFile=C:\Documents\Документация\J1939\j1939.dbc  MsgList=A1  MsgName=CANPACK  MsgIDType=Extended (29-bit identifier)  MsgIdentifier=hex2dec('18FEFB10')  MsgLength=8  Remote=off  ApplyMinMax=off  BusOutput=off  SignalInfo={ 'ActualEngPercentTorque', '16', '8', 'LE', 'unsigned', 'Standard', '0', '1', '-125', '-125', '125'; 'DriversDemandEngPercentTorque', '8', '8', 'LE', 'unsigned', 'Standard', '0', '1', '-125', '-125', '125'; 'EngDemandPercentTorque', '56', '8', 'LE', 'unsigned', 'Standard', '0', '1', '-125', '-125', '125'; 'EngSpeed', '24', '16', 'LE', 'unsigned', 'Standard', '0', '0.125', '0', '0', '8031.875'; 'EngStarterMode', '48', '4', 'LE', 'unsigned', 'Standard', '0', '1', '0', '0', '15'; 'EngTorqueMode', '0', '4', 'LE', 'unsigned', 'Standard', '0', '1', '0', '0', '15'; 'SrcAddrssOfCtrllngDvcForEngCtrl', '40', '8', 'LE', 'unsigned', 'Standard', '0', '1', '0', '0', '255' }
      settings: SourceProductBaseCode=ME,XP,VN  DataFormat=raw data
  CAN Unpack8 : canmsglib/CAN Unpack  CANdbFile=C:\Users\km-rta\Desktop\engineering\j1939.dbc  MsgList=RF  MsgName=RF  MsgIDType=Extended (29-bit identifier)  MsgIdentifier=hex2dec('18FEFB10')  MsgLength=8  SignalInfo={ 'HydRetarderOilTemp', '8', '8', 'LE', 'unsigned', 'Standard', '0', '1', '-40', '-40', '210' }  IDPort=off  TimestampPort=off  ErrorPort=off  RemotePort=off  LengthPort=off  StatusPort=off  ApplyMinMax=off
      settings: SourceProductName=Simulink Real-Time
  Constant : Constant  Value=0  OutDataTypeStr=uint16
  Data Store Write : DataStoreWrite  DataStoreName=ret  DataStoreElements=ret.RetTemp  IndexOptions=Index vector (dialog)  Indices=1  OutputSizes=1
  Data Store Write1 : DataStoreWrite  DataStoreName=wtdg_CAN  DataStoreElements=wtdg_CAN.RF  IndexOptions=Index vector (dialog)  Indices=1  OutputSizes=1
  wires:
  CAN Pack/1 -> CAN Unpack8/1
  Data/1 -> CAN Pack/1
  CAN Unpack8/1 -> Data Store Write/1
  Constant/1 -> Data Store Write1/1

== system BCM2_4/CAN_Receive/RX_FIFO_Complete_Event buf 0-4/VD 0x18FEE000 buf = 1 ==
  Data : Inport
  Action Port : ActionPort  ActionPortLabel=case [ 419356672 ]:
  CAN Pack : canmsglib/CAN Pack  CANdbFile=C:\Documents\Документация\J1939\j1939.dbc  MsgList=A1  MsgName=CANPACK  MsgIDType=Extended (29-bit identifier)  MsgIdentifier=hex2dec('18FEE000')  MsgLength=8  Remote=off  ApplyMinMax=off  BusOutput=off  SignalInfo={ 'ActualEngPercentTorque', '16', '8', 'LE', 'unsigned', 'Standard', '0', '1', '-125', '-125', '125'; 'DriversDemandEngPercentTorque', '8', '8', 'LE', 'unsigned', 'Standard', '0', '1', '-125', '-125', '125'; 'EngDemandPercentTorque', '56', '8', 'LE', 'unsigned', 'Standard', '0', '1', '-125', '-125', '125'; 'EngSpeed', '24', '16', 'LE', 'unsigned', 'Standard', '0', '0.125', '0', '0', '8031.875'; 'EngStarterMode', '48', '4', 'LE', 'unsigned', 'Standard', '0', '1', '0', '0', '15'; 'EngTorqueMode', '0', '4', 'LE', 'unsigned', 'Standard', '0', '1', '0', '0', '15'; 'SrcAddrssOfCtrllngDvcForEngCtrl', '40', '8', 'LE', 'unsigned', 'Standard', '0', '1', '0', '0', '255' }
      settings: SourceProductBaseCode=ME,XP,VN  DataFormat=raw data
  CAN Unpack5 : canmsglib/CAN Unpack  CANdbFile=C:\Users\km-rta\Desktop\engineering\j1939.dbc  MsgList=VD  MsgName=VD  MsgIDType=Extended (29-bit identifier)  MsgIdentifier=hex2dec('18FEE000')  MsgLength=8  SignalInfo={ 'TripDistance', '0', '32', 'LE', 'unsigned', 'Standard', '0', '0.125', '0', '0', '526385151.9' }  IDPort=off  TimestampPort=off  ErrorPort=off  RemotePort=off  LengthPort=off  StatusPort=off  ApplyMinMax=off
      settings: SourceProductBaseCode=ME,XP,VN
  Constant : Constant  Value=0  OutDataTypeStr=uint16
  Data Store Write : DataStoreWrite  DataStoreName=CAN_rec  DataStoreElements=CAN_rec.total_dist  IndexOptions=Index vector (dialog)  Indices=1  OutputSizes=1
  Data Store Write1 : DataStoreWrite  DataStoreName=wtdg_CAN  DataStoreElements=wtdg_CAN.VD  IndexOptions=Index vector (dialog)  Indices=1  OutputSizes=1
  wires:
  Constant/1 -> Data Store Write1/1
  CAN Unpack5/1 -> Data Store Write/1
  CAN Pack/1 -> CAN Unpack5/1
  Data/1 -> CAN Pack/1

== system BCM2_4/CAN_Receive/RX_FIFO_Complete_Event buf 0-4/кнопки на руле 0х1FEEF888 buf = 3 ==
  Data : Inport
  Action Port : ActionPort  ActionPortLabel=case [ 535754888 ]:
  CAN Pack : canmsglib/CAN Pack  CANdbFile=C:\Documents\Документация\J1939\j1939.dbc  MsgList=A1  MsgName=CANPACK  MsgIDType=Extended (29-bit identifier)  MsgIdentifier=hex2dec('1FEEF888')  MsgLength=8  Remote=off  ApplyMinMax=off  BusOutput=off  SignalInfo={ 'ActualEngPercentTorque', '16', '8', 'LE', 'unsigned', 'Standard', '0', '1', '-125', '-125', '125'; 'DriversDemandEngPercentTorque', '8', '8', 'LE', 'unsigned', 'Standard', '0', '1', '-125', '-125', '125'; 'EngDemandPercentTorque', '56', '8', 'LE', 'unsigned', 'Standard', '0', '1', '-125', '-125', '125'; 'EngSpeed', '24', '16', 'LE', 'unsigned', 'Standard', '0', '0.125', '0', '0', '8031.875'; 'EngStarterMode', '48', '4', 'LE', 'unsigned', 'Standard', '0', '1', '0', '0', '15'; 'EngTorqueMode', '0', '4', 'LE', 'unsigned', 'Standard', '0', '1', '0', '0', '15'; 'SrcAddrssOfCtrllngDvcForEngCtrl', '40', '8', 'LE', 'unsigned', 'Standard', '0', '1', '0', '0', '255' }
      settings: SourceProductBaseCode=ME,XP,VN  DataFormat=raw data
  CAN Unpack5 : canmsglib/CAN Unpack  CANdbFile=C:\Users\km-rta\Desktop\engineering\j1939.dbc  MsgList=A1  MsgName=Wireless_buttons  MsgIDType=Extended (29-bit identifier)  MsgIdentifier=hex2dec('1FEEF888')  MsgLength=8  SignalInfo={ 'but_cmd', '0', '8', 'LE', 'unsigned', 'Standard', '0', '1', '0', '-Inf', 'Inf'; 'channel', '8', '8', 'LE', 'unsigned', 'Standard', '0', '1', '0', '-Inf', 'Inf' }  IDPort=off  TimestampPort=off  ErrorPort=off  RemotePort=off  LengthPort=off  StatusPort=off  ApplyMinMax=off
      settings: SourceProductBaseCode=ME,XP,VN
  Constant : Constant  Value=0  OutDataTypeStr=uint16
  Data Store Write : DataStoreWrite  DataStoreName=CAN_rec  DataStoreElements=CAN_rec.wireless_chan  IndexOptions=Index vector (dialog)  Indices=1  OutputSizes=1
  Data Store Write1 : DataStoreWrite  DataStoreName=wtdg_CAN  DataStoreElements=wtdg_CAN.wireless_chan  IndexOptions=Index vector (dialog)  Indices=1  OutputSizes=1
  Terminator : Terminator
  wires:
  Constant/1 -> Data Store Write1/1
  CAN Pack/1 -> CAN Unpack5/1
  Data/1 -> CAN Pack/1
  CAN Unpack5/2 -> Data Store Write/1
  CAN Unpack5/1 -> Terminator/1

== system BCM2_4/CAN_Receive/RX_FIFO_Complete_Event buf 0-4/страницы пилот 0х181112F3 buf = 2 ==
  Data : Inport
  Action Port : ActionPort  ActionPortLabel=case [ 403772147 ]:
  CAN Pack : canmsglib/CAN Pack  CANdbFile=C:\Documents\Документация\J1939\j1939.dbc  MsgList=A1  MsgName=CANPACK  MsgIDType=Extended (29-bit identifier)  MsgIdentifier=hex2dec('181112F3')  MsgLength=8  Remote=off  ApplyMinMax=off  BusOutput=off  SignalInfo={ 'ActualEngPercentTorque', '16', '8', 'LE', 'unsigned', 'Standard', '0', '1', '-125', '-125', '125'; 'DriversDemandEngPercentTorque', '8', '8', 'LE', 'unsigned', 'Standard', '0', '1', '-125', '-125', '125'; 'EngDemandPercentTorque', '56', '8', 'LE', 'unsigned', 'Standard', '0', '1', '-125', '-125', '125'; 'EngSpeed', '24', '16', 'LE', 'unsigned', 'Standard', '0', '0.125', '0', '0', '8031.875'; 'EngStarterMode', '48', '4', 'LE', 'unsigned', 'Standard', '0', '1', '0', '0', '15'; 'EngTorqueMode', '0', '4', 'LE', 'unsigned', 'Standard', '0', '1', '0', '0', '15'; 'SrcAddrssOfCtrllngDvcForEngCtrl', '40', '8', 'LE', 'unsigned', 'Standard', '0', '1', '0', '0', '255' }
      settings: SourceProductBaseCode=ME,XP,VN  DataFormat=raw data
  CAN Unpack5 : canmsglib/CAN Unpack  CANdbFile=C:\Users\km-rta\Desktop\engineering\j1939.dbc  MsgList=A1  MsgName=Fuel_tank  MsgIDType=Extended (29-bit identifier)  MsgIdentifier=hex2dec('181112F3')  MsgLength=8  SignalInfo={ 'max_page', '8', '8', 'LE', 'unsigned', 'Standard', '0', '1', '0', '-Inf', 'Inf' }  IDPort=off  TimestampPort=off  ErrorPort=off  RemotePort=off  LengthPort=off  StatusPort=off  ApplyMinMax=off
      settings: SourceProductBaseCode=ME,XP,VN
  Constant : Constant  Value=0  OutDataTypeStr=uint16
  Data Store Write : DataStoreWrite  DataStoreName=disp  DataStoreElements=disp.pilot_max_page  IndexOptions=Index vector (dialog)  Indices=1  OutputSizes=1
  Data Store Write1 : DataStoreWrite  DataStoreName=wtdg_CAN  DataStoreElements=wtdg_CAN.max_page_pilot  IndexOptions=Index vector (dialog)  Indices=1  OutputSizes=1
  wires:
  Constant/1 -> Data Store Write1/1
  CAN Unpack5/1 -> Data Store Write/1
  CAN Pack/1 -> CAN Unpack5/1
  Data/1 -> CAN Pack/1

== system BCM2_4/CAN_Receive/RX_FIFO_Complete_Event buf 0-4/страницы пилот 0х181112F5 buf = 2 ==
  Data : Inport
  Action Port : ActionPort  ActionPortLabel=case [ 403772149 ]:
  CAN Pack : canmsglib/CAN Pack  CANdbFile=C:\Documents\Документация\J1939\j1939.dbc  MsgList=A1  MsgName=CANPACK  MsgIDType=Extended (29-bit identifier)  MsgIdentifier=hex2dec('181112F5')  MsgLength=8  Remote=off  ApplyMinMax=off  BusOutput=off  SignalInfo={ 'ActualEngPercentTorque', '16', '8', 'LE', 'unsigned', 'Standard', '0', '1', '-125', '-125', '125'; 'DriversDemandEngPercentTorque', '8', '8', 'LE', 'unsigned', 'Standard', '0', '1', '-125', '-125', '125'; 'EngDemandPercentTorque', '56', '8', 'LE', 'unsigned', 'Standard', '0', '1', '-125', '-125', '125'; 'EngSpeed', '24', '16', 'LE', 'unsigned', 'Standard', '0', '0.125', '0', '0', '8031.875'; 'EngStarterMode', '48', '4', 'LE', 'unsigned', 'Standard', '0', '1', '0', '0', '15'; 'EngTorqueMode', '0', '4', 'LE', 'unsigned', 'Standard', '0', '1', '0', '0', '15'; 'SrcAddrssOfCtrllngDvcForEngCtrl', '40', '8', 'LE', 'unsigned', 'Standard', '0', '1', '0', '0', '255' }
      settings: SourceProductBaseCode=ME,XP,VN  DataFormat=raw data
  CAN Unpack5 : canmsglib/CAN Unpack  CANdbFile=C:\Users\km-rta\Desktop\engineering\j1939.dbc  MsgList=A1  MsgName=Fuel_tank  MsgIDType=Extended (29-bit identifier)  MsgIdentifier=hex2dec('181112F5')  MsgLength=8  SignalInfo={ 'max_page', '8', '8', 'LE', 'unsigned', 'Standard', '0', '1', '0', '-Inf', 'Inf' }  IDPort=off  TimestampPort=off  ErrorPort=off  RemotePort=off  LengthPort=off  StatusPort=off  ApplyMinMax=off
      settings: SourceProductBaseCode=ME,XP,VN
  Constant : Constant  Value=0  OutDataTypeStr=uint16
  Data Store Write : DataStoreWrite  DataStoreName=disp  DataStoreElements=disp.meh_max_page  IndexOptions=Index vector (dialog)  Indices=1  OutputSizes=1
  Data Store Write1 : DataStoreWrite  DataStoreName=wtdg_CAN  DataStoreElements=wtdg_CAN.max_page_meh  IndexOptions=Index vector (dialog)  Indices=1  OutputSizes=1
  wires:
  Data/1 -> CAN Pack/1
  CAN Pack/1 -> CAN Unpack5/1
  CAN Unpack5/1 -> Data Store Write/1
  Constant/1 -> Data Store Write1/1

== system BCM2_4/CAN_Receive/RX_FIFO_Complete_Event buf 0-4/уровень топлива 0х18FEFC01 buf = 1 ==
  Data : Inport
  Action Port : ActionPort  ActionPortLabel=case [ 419363841 ]:
  CAN Pack : canmsglib/CAN Pack  CANdbFile=C:\Documents\Документация\J1939\j1939.dbc  MsgList=A1  MsgName=CANPACK  MsgIDType=Extended (29-bit identifier)  MsgIdentifier=hex2dec('18FEFC01')  MsgLength=8  Remote=off  ApplyMinMax=off  BusOutput=off  SignalInfo={ 'ActualEngPercentTorque', '16', '8', 'LE', 'unsigned', 'Standard', '0', '1', '-125', '-125', '125'; 'DriversDemandEngPercentTorque', '8', '8', 'LE', 'unsigned', 'Standard', '0', '1', '-125', '-125', '125'; 'EngDemandPercentTorque', '56', '8', 'LE', 'unsigned', 'Standard', '0', '1', '-125', '-125', '125'; 'EngSpeed', '24', '16', 'LE', 'unsigned', 'Standard', '0', '0.125', '0', '0', '8031.875'; 'EngStarterMode', '48', '4', 'LE', 'unsigned', 'Standard', '0', '1', '0', '0', '15'; 'EngTorqueMode', '0', '4', 'LE', 'unsigned', 'Standard', '0', '1', '0', '0', '15'; 'SrcAddrssOfCtrllngDvcForEngCtrl', '40', '8', 'LE', 'unsigned', 'Standard', '0', '1', '0', '0', '255' }
      settings: SourceProductBaseCode=ME,XP,VN  DataFormat=raw data
  CAN Unpack5 : canmsglib/CAN Unpack  CANdbFile=C:\Users\km-rta\Desktop\engineering\j1939.dbc  MsgList=A1  MsgName=Fuel_tank  MsgIDType=Extended (29-bit identifier)  MsgIdentifier=hex2dec('18FEFC01')  MsgLength=8  SignalInfo={ 'Tank1', '0', '16', 'LE', 'unsigned', 'Standard', '0', '1', '0', '-Inf', 'Inf'; 'Tank2', '16', '16', 'LE', 'unsigned', 'Standard', '0', '1', '0', '-Inf', 'Inf'; 'Tank3', '32', '16', 'LE', 'unsigned', 'Standard', '0', '1', '0', '-Inf', 'Inf' }  IDPort=off  TimestampPort=off  ErrorPort=off  RemotePort=off  LengthPort=off  StatusPort=off  ApplyMinMax=off
      settings: SourceProductBaseCode=ME,XP,VN
  Constant : Constant  Value=0  OutDataTypeStr=uint16
  Data Store Write : DataStoreWrite  DataStoreName=CAN_rec  DataStoreElements=CAN_rec.FuelTank1#CAN_rec.FuelTank2#CAN_rec.FuelTank3  IndexOptions=Index vector (dialog)  Indices=1  OutputSizes=1
  Data Store Write1 : DataStoreWrite  DataStoreName=wtdg_CAN  DataStoreElements=wtdg_CAN.FuelTank  IndexOptions=Index vector (dialog)  Indices=1  OutputSizes=1
  wires:
  Data/1 -> CAN Pack/1
  CAN Pack/1 -> CAN Unpack5/1
  CAN Unpack5/1 -> Data Store Write/1
  Constant/1 -> Data Store Write1/1
  CAN Unpack5/2 -> Data Store Write/2
  CAN Unpack5/3 -> Data Store Write/3

== system BCM2_4/CAN_Receive/RX_FIFO_Complete_Event2 buf 22-26/ID0X101 buf = 22 ==
  Data : Inport
  Action Port : ActionPort  ActionPortLabel=case [ 257 ]:
  CAN Pack1 : canmsglib/CAN Pack  CANdbFile=C:\Documents\Документация\J1939\j1939.dbc  MsgList=A1  MsgName=CANPACK  MsgIDType=Standard (11-bit identifier)  MsgIdentifier=hex2dec('101')  MsgLength=8  Remote=off  ApplyMinMax=off  BusOutput=off  SignalInfo={}
      settings: SourceProductBaseCode=ME,XP,VN  DataFormat=raw data
  CAN Unpack1 : canmsglib/CAN Unpack  MsgList=(none)  MsgName=ASU  MsgIDType=Standard (11-bit identifier)  MsgIdentifier="hex2dec(\"101\")"  MsgLength=8  SignalInfo={ 'buttons', '0', '16', 'LE', 'unsigned', 'Standard', '0', '1', '0', '0', 'inf' }  IDPort=off  TimestampPort=off  ErrorPort=off  RemotePort=off  LengthPort=off  StatusPort=off  ApplyMinMax=off
      settings: SourceProductName=Simulink Real-Time
  Constant : Constant  Value=0  OutDataTypeStr=uint16
  Data Store Write1 : DataStoreWrite  DataStoreName=wtdg_CAN  DataStoreElements=wtdg_CAN.id101  IndexOptions=Index vector (dialog)  Indices=1  OutputSizes=1
  Terminator : Terminator
  wires:
  Constant/1 -> Data Store Write1/1
  Data/1 -> CAN Pack1/1
  CAN Pack1/1 -> CAN Unpack1/1
  CAN Unpack1/1 -> Terminator/1

== system BCM2_4/CAN_Receive/RX_FIFO_Complete_Event2 buf 22-26/ID0X18F0010B buf = 23 ==
  Data : Inport
  Action Port : ActionPort  ActionPortLabel=case [ 418382091 ]:
  Constant : Constant  Value=0  OutDataTypeStr=uint16
  Data Store Write1 : DataStoreWrite  DataStoreName=wtdg_CAN  DataStoreElements=wtdg_CAN.w18F0010B  IndexOptions=Index vector (dialog)  Indices=1  OutputSizes=1
  Data Store Write2 : DataStoreWrite  DataStoreName=CAN_rec  DataStoreElements=CAN_rec.m18F0010B(:)  IndexOptions=Index vector (dialog)  Indices=1  OutputSizes=1
  wires:
  Constant/1 -> Data Store Write1/1
  Data/1 -> Data Store Write2/1

== system BCM2_4/CAN_Receive/RX_FIFO_Complete_Event2 buf 22-26/ID0X18FEAD0B buf = 23 ==
  Data : Inport
  Action Port : ActionPort  ActionPortLabel=case [ 419343627 ]:
  Constant : Constant  Value=0  OutDataTypeStr=uint16
  Data Store Write1 : DataStoreWrite  DataStoreName=wtdg_CAN  DataStoreElements=wtdg_CAN.w18FEAD0B  IndexOptions=Index vector (dialog)  Indices=1  OutputSizes=1
  Data Store Write2 : DataStoreWrite  DataStoreName=CAN_rec  DataStoreElements=CAN_rec.m18FEAD0B(:)  IndexOptions=Index vector (dialog)  Indices=1  OutputSizes=1
  wires:
  Data/1 -> Data Store Write2/1
  Constant/1 -> Data Store Write1/1
